simulink model "SimplePendulumMotion"  (R2023a)
settings: Solver=VariableStepAuto  StartTime=0.0  StopTime=10.0  MaxStep=1e-3  RelTol=1e-3
settings Model: Creator=eslam  LastModifiedBy=eslam

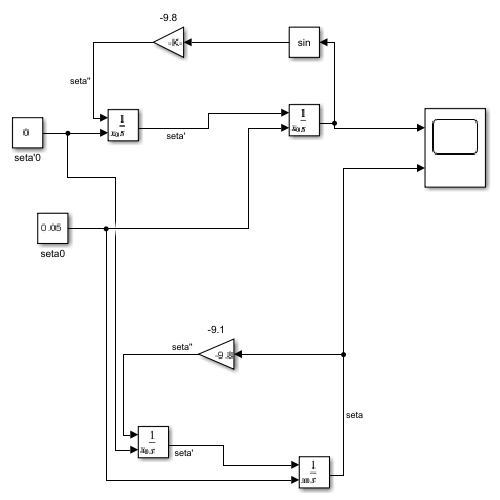
[thumbnail: Simulink's stored preview of the top-level diagram]
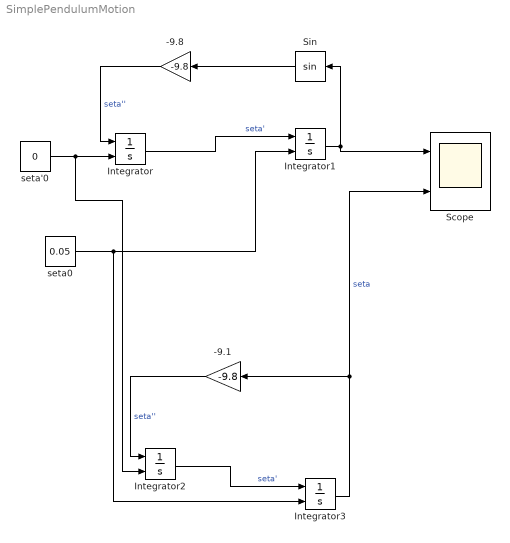
== system SimplePendulumMotion ==
  -9.1 : Gain  Gain=-9.8
  -9.8 : Gain  Gain=-9.8
  Integrator{,1..3} (4 alike) : Integrator  InitialConditionSource=external
  Scope : Scope  NumInputPorts=2
  Sin : Trigonometry
  seta'0 : Constant  Value=0
  seta0 : Constant  Value=0.05
  wires:
  Integrator/1 -> Integrator1/1  "seta'"
  -9.8/1 -> Integrator/1  "seta''"
  seta'0/1 -> Integrator2/2, Integrator/2
  Sin/1 -> -9.8/1
  Integrator1/1 -> Scope/1, Sin/1
  seta0/1 -> Integrator3/2, Integrator1/2
  Integrator2/1 -> Integrator3/1  "seta'"
  -9.1/1 -> Integrator2/1  "seta''"
  Integrator3/1 -> Scope/2, -9.1/1  "seta"
